simulink model "Highway_Assistant"  (R2023b)
settings: Solver=FixedStepDiscrete  StartTime=0.0  StopTime=10.0  FixedStep=0.01  RelTol=1e-3
settings Model: DataDictionary=Highway_Assistant.sldd  Creator=Shoyab Silar  LastModifiedBy=Shoyab Silar
settings DataIOCC: SaveFormat=StructureWithTime
settings OptimizationCC: DefaultParameterBehavior=Inlined  EnhancedBackFolding=on  PassReuseOutputArgsAs=Individual arguments  ZeroExternalMemoryAtStartup=off  ZeroInternalMemoryAtStartup=off  OptimizeBlockOrder=speed  DifferentSizesBufferReuse=on  OptimizationCustomize=off  EfficientTunableParamExpr=on
settings DebuggingCC: ParameterTunabilityLossMsg=error
settings SFSimCC: MATLABDynamicMemAlloc=off
settings RTWCC: Description=AUTOSAR  SystemTargetFile=autosar.tlc  GenCodeOnly=on  TemplateMakefile=ert_default_tmf  DataTypeReplacement=CDataTypesFixedWidth
settings CodeAppCC: ForceParamTrailComments=on  IgnoreCustomStorageClasses=off  OperatorAnnotations=on  SimulinkDataObjDesc=on  SFDataObjDesc=on  InsertBlockDesc=on
settings STFCustomTargetCC: MultiwordLength=256  ParMdlRefBuildCompliant=on  CompOptLevelCompliant=on  IncludeMdlTerminateFcn=off  CombineOutputUpdateFcns=on  SuppressErrorStatus=on  ERTCustomFileBanners=on  SupportNonFinite=off  SupportComplex=off  SupportContinuousTime=off  SupportNonInlinedSFcns=off  RemoveResetFunc=on  MATLABClassNameForMDSCustomization=Simulink.SoftwareTarget.ERTCustomization  AutosarCompliant=on  UseToolchainInfoCompliant=on  LookupTableObjectStructAxisOrder=2,1,3,4,...  LUTObjectStructOrderEvenSpacing=Size,Table,Breakpoints  SystemTargetFile=autosar.tlc
settings ERTTargetCC: TargetLangStandard=C99 (ISO)  ConcurrentExecutionCompliant=off  IncludeMdlTerminateFcn=off  SuppressErrorStatus=on  SupportNonFinite=off  SupportComplex=off  ModelStepFunctionPrototypeControlCompliant=off  CPPClassGenCompliant=off  AutosarCompliant=on  LookupTableObjectStructAxisOrder=2,1,3,4,...  LUTObjectStructOrderEvenSpacing=Size,Table,Breakpoints  InlinedParameterPlacement=NonHierarchical  ERTCustomFileTemplate=example_file_process.tlc  BooleanTrueId=TRUE  BooleanFalseId=FALSE

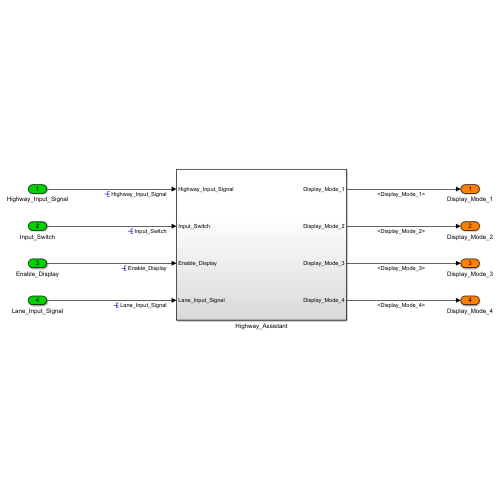
[thumbnail: Simulink's stored preview of the top-level diagram]
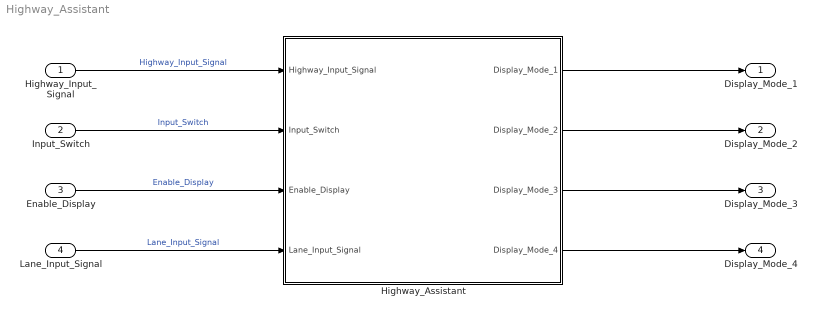
== system Highway_Assistant ==
  Highway_Input_Signal : Inport  OutMin=0  OutMax=255  OutDataTypeStr=uint8  PortDimensions=1
  Input_Switch : Inport  Port=2  OutMin=0  OutMax=255  OutDataTypeStr=uint8  PortDimensions=1
  Enable_Display : Inport  Port=3  OutMin=0  OutMax=255  OutDataTypeStr=uint8  PortDimensions=1
  Lane_Input_Signal : Inport  Port=4  OutMin=0  OutMax=255  OutDataTypeStr=uint8  PortDimensions=1
  Highway_Assistant : Subsystem
  Display_Mode_1 : Outport
  Display_Mode_2 : Outport  Port=2
  Display_Mode_3 : Outport  Port=3
  Display_Mode_4 : Outport  Port=4
  wires:
  Input_Switch/1 -> Highway_Assistant/2(Input_Switch)  "Input_Switch"
  Enable_Display/1 -> Highway_Assistant/3(Enable_Display)  "Enable_Display"
  Highway_Input_Signal/1 -> Highway_Assistant/1(Highway_Input_Signal)  "Highway_Input_Signal"
  Lane_Input_Signal/1 -> Highway_Assistant/4(Lane_Input_Signal)  "Lane_Input_Signal"
  Highway_Assistant/1(Display_Mode_1) -> Display_Mode_1/1
  Highway_Assistant/2(Display_Mode_2) -> Display_Mode_2/1
  Highway_Assistant/3(Display_Mode_3) -> Display_Mode_3/1
  Highway_Assistant/4(Display_Mode_4) -> Display_Mode_4/1

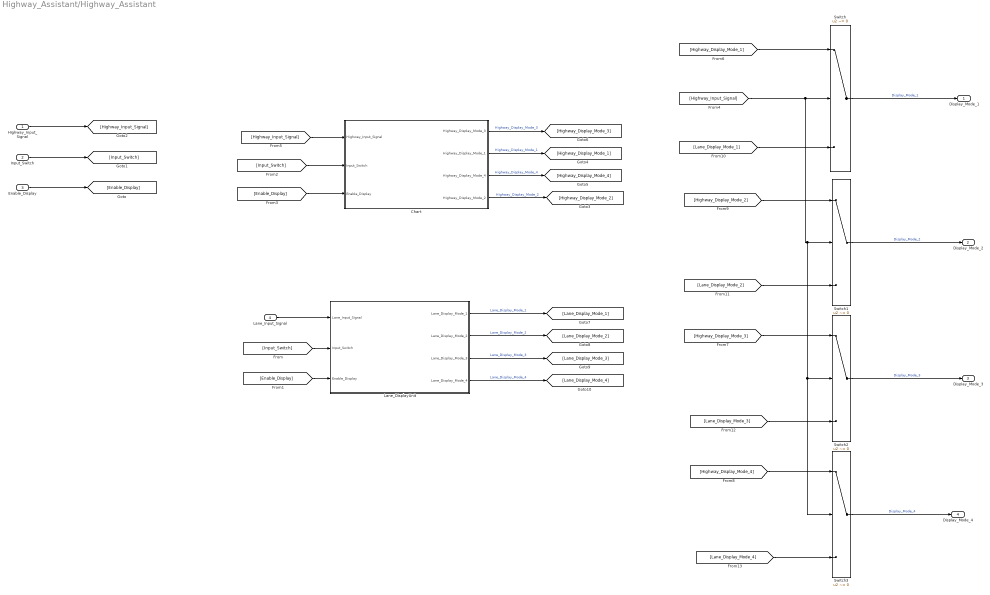
== system Highway_Assistant/Highway_Assistant ==
  Highway_Input_Signal : Inport  OutDataTypeStr=uint8  PortDimensions=1
  Input_Switch : Inport  Port=2  OutDataTypeStr=uint8  PortDimensions=1
  Enable_Display : Inport  Port=3  OutMin=0  OutMax=255  OutDataTypeStr=uint8  PortDimensions=1
  Lane_Input_Signal : Inport  Port=4  OutDataTypeStr=uint8  PortDimensions=1
  Chart : Stateflow chart  TreatAsAtomicUnit=on
  Lane_DisplayUnit : Stateflow chart  TreatAsAtomicUnit=on
  Switch{,1..3} (4 alike) : Switch  Criteria=u2 ~= 0  SaturateOnIntegerOverflow=off  InputSameDT=off
  Display_Mode_1 : Outport
  Display_Mode_2 : Outport  Port=2
  Display_Mode_3 : Outport  Port=3
  Display_Mode_4 : Outport  Port=4
  wires:
  Enable_Display/1 -> [Enable_Display]
  Input_Switch/1 -> [Input_Switch]
  Lane_Input_Signal/1 -> Lane_DisplayUnit/1(Lane_Input_Signal)
  Highway_Input_Signal/1 -> [Highway_Input_Signal]
  [Highway_Input_Signal] -> Switch/2, Switch3/2, Switch2/2, Switch1/2
  [Enable_Display] -> Lane_DisplayUnit/3(Enable_Display)
  [Input_Switch] -> Lane_DisplayUnit/2(Input_Switch)
  [Highway_Input_Signal] -> Chart/1(Highway_Input_Signal)
  [Input_Switch] -> Chart/2(Input_Switch)
  [Enable_Display] -> Chart/3(Enable_Display)
  Switch/1 -> Display_Mode_1/1  "Display_Mode_1"
  Switch3/1 -> Display_Mode_4/1  "Display_Mode_4"
  Switch1/1 -> Display_Mode_2/1  "Display_Mode_2"
  Switch2/1 -> Display_Mode_3/1  "Display_Mode_3"
  Chart/2(Highway_Display_Mode_1) -> [Highway_Display_Mode_1]  "Highway_Display_Mode_1"
  Chart/4(Highway_Display_Mode_2) -> [Highway_Display_Mode_2]  "Highway_Display_Mode_2"
  Chart/1(Highway_Display_Mode_3) -> [Highway_Display_Mode_3]  "Highway_Display_Mode_3"
  Chart/3(Highway_Display_Mode_4) -> [Highway_Display_Mode_4]  "Highway_Display_Mode_4"
  Lane_DisplayUnit/1(Lane_Display_Mode_1) -> [Lane_Display_Mode_1]  "Lane_Display_Mode_1"
  Lane_DisplayUnit/2(Lane_Display_Mode_2) -> [Lane_Display_Mode_2]  "Lane_Display_Mode_2"
  Lane_DisplayUnit/3(Lane_Display_Mode_3) -> [Lane_Display_Mode_3]  "Lane_Display_Mode_3"
  Lane_DisplayUnit/4(Lane_Display_Mode_4) -> [Lane_Display_Mode_4]  "Lane_Display_Mode_4"
  [Highway_Display_Mode_1] -> Switch/1
  [Lane_Display_Mode_1] -> Switch/3
  [Lane_Display_Mode_2] -> Switch1/3
  [Highway_Display_Mode_2] -> Switch1/1
  [Highway_Display_Mode_3] -> Switch2/1
  [Lane_Display_Mode_3] -> Switch2/3
  [Highway_Display_Mode_4] -> Switch3/1
  [Lane_Display_Mode_4] -> Switch3/3

== stateflow chart Highway_Assistant/Chart ==
  state Default
    Highway_Display_Mode_1 = 0;
    Highway_Display_Mode_2 = 0;
    Highway_Display_Mode_3 = 0;
    Highway_Display_Mode_4 = 0;
  state HW_Mode_ON_
    Highway_Display_Mode_1 = 213;
    Highway_Display_Mode_2 = 183;
    Highway_Display_Mode_3 = 9;
    Highway_Display_Mode_4 = 94;
  state HW_Mode_OFF_
    Highway_Display_Mode_1 = 232;
    Highway_Display_Mode_2 = 183;
    Highway_Display_Mode_3 = 41;
    Highway_Display_Mode_4 = 94;
  (default) -> Default
  Default -> HW_Mode_OFF_ [order 1] : [Highway_Input_Signal == 1 && Enable_Display == 0 && Input_Switch == 1]
  Default -> HW_Mode_ON_ [order 2] : [Highway_Input_Signal == 1 && Enable_Display == 1 && Input_Switch == 1]
  HW_Mode_OFF_ -> HW_Mode_ON_ [order 1] : [Enable_Display == 1]
  HW_Mode_ON_ -> HW_Mode_OFF_ [order 1] : [Enable_Display == 0]
  HW_Mode_ON_ -> (junction 6) [order 2]
  HW_Mode_OFF_ -> (junction 5) [order 2]
  data: Highway_Display_Mode_3 output uint8; Highway_Input_Signal input; Input_Switch input; Enable_Display input; Highway_Display_Mode_1 output uint8; Highway_Display_Mode_4 output uint8; Highway_Display_Mode_2 output uint8

== stateflow chart Highway_Assistant/Lane_DisplayUnit ==
  state Default
    Lane_Display_Mode_1 = 0;
    Lane_Display_Mode_2 = 0;
    Lane_Display_Mode_3 = 0;
    Lane_Display_Mode_4 = 0;
  note: [Lane_Input_Signal == 6 && Enable_Display == 1 && Input_Switch == 1]
  state Lane_Mode_ON
    Lane_Display_Mode_1 = 127;
    Lane_Display_Mode_2 = 248;
    Lane_Display_Mode_3 = 186;
    Lane_Display_Mode_4 = 84;
  state Lane_Mode_OFF
    Lane_Display_Mode_1 = 132;
    Lane_Display_Mode_2 = 185;
    Lane_Display_Mode_3 = 54;
    Lane_Display_Mode_4 = 67;
  (default) -> Default
  Default -> state1 [order 1] : [Lane_Input_Signal == 6 && Enable_Display == 0 && Input_Switch == 1]
  Default -> state4 [order 2]
  state1 -> state4 [order 1] : [Enable_Display == 1]
  state4 -> state1 [order 1] : [Enable_Display == 0]
  state1 -> (junction 15) [order 2]
  state4 -> (junction 5) [order 2]
  data: Lane_Input_Signal input uint8; Input_Switch input uint8; Lane_Display_Mode_1 output uint8; Lane_Display_Mode_2 output uint8; Lane_Display_Mode_3 output uint8; Enable_Display input uint8; Lane_Display_Mode_4 output uint8
